simulink model "ball"  (R2020a)
settings: Solver=VariableStepAuto  StartTime=0.0  StopTime=10.0  RelTol=1e-3
undefined symbols (not defined in the file): d, g, J, L, m, R
settings Model: Creator=Mike  LastModifiedBy=Mike

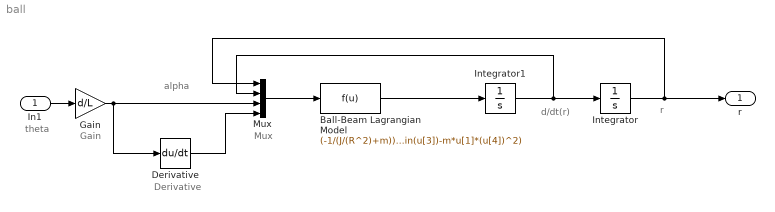
== system ball ==
  note: Gain
  note: theta
  note: Mux
  note: Derivative
  note: alpha
  note: r
  note: d/dt(r)
  In1 : Inport
  Ball-Beam Lagrangian Model : Fcn  Expr=(-1/(J/(R^2)+m))*(m*g*sin(u[3])-m*u[1]*(u[4])^2)
  Derivative : Derivative
  Gain : Gain  Gain=d/L
  Integrator : Integrator
  Integrator1 : Integrator
  Mux : Mux
  r : Outport
  wires:
  Integrator1/1 -> Mux/2, Integrator/1
  Integrator/1 -> Mux/1, r/1
  Ball-Beam Lagrangian Model/1 -> Integrator1/1
  Mux/1 -> Ball-Beam Lagrangian Model/1
  In1/1 -> Gain/1
  Gain/1 -> Derivative/1, Mux/3
  Derivative/1 -> Mux/4
